simulink model "Part1"  (R2021a)
settings: Solver=VariableStepAuto  StartTime=0.0  StopTime=10.0  RelTol=1e-3
model workspace (MAT data in the model file):
  d = 0.003
settings Model: Creator=legen  LastModifiedBy=legen

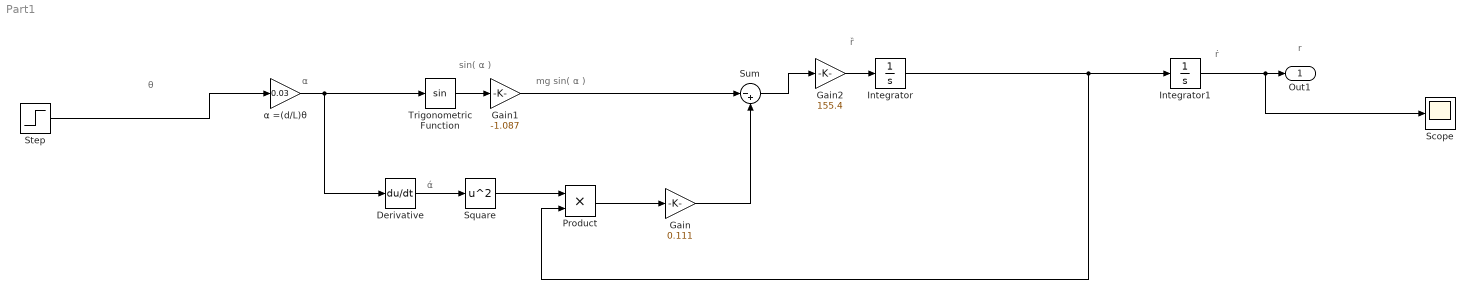
== system Part1 ==
  note: ṙ
  note: ȑ
  note: sin( α )
  note: ά
  note: α
  note: r
  note: θ
  note: mg sin( α )
  Derivative : Derivative
  Gain : Gain  Gain=0.111
  Gain1 : Gain  Gain=-1.087
  Gain2 : Gain  Gain=155.4
  Integrator : Integrator
  Integrator1 : Integrator
  Product : Product
  Scope : Scope
  Square : Math  Operator=square  SaturateOnIntegerOverflow=on
  Step : Step  Time=0  SampleTime=0
  Sum : Sum  Inputs=|-+
  Trigonometric Function : Trigonometry
  "α =(d/L)θ " : Gain  Gain=0.03
  Out1 : Outport
  wires:
  Integrator1/1 -> Scope/1, Out1/1
  "α =(d/L)θ "/1 -> Trigonometric Function/1, Derivative/1
  Trigonometric Function/1 -> Gain1/1
  Gain1/1 -> Sum/1
  Gain2/1 -> Integrator/1
  Sum/1 -> Gain2/1
  Derivative/1 -> Square/1
  Gain/1 -> Sum/2
  Product/1 -> Gain/1
  Square/1 -> Product/1
  Integrator/1 -> Product/2, Integrator1/1
  Step/1 -> "α =(d/L)θ "/1
